simulink model "sm_DynamicCompressionOLD"  (R2019a)
settings: Solver=FixedStepDiscrete  StartTime=0.0  StopTime=stop_time  RelTol=1e-3
InitFcn:
  | sm_callback_init
StopFcn:
  | sm_callback_stop
values from neighbouring files (symbols this model uses):
  calib_bpfs = bpfs    [sm_compression_init.m]
  delayFix = maxDelay-delays    [Initialize_Delay_Values.m]
  F_bits = 28    [TestingLibraryScripts.m]    (also in sm_compression_init.m)
  M_bits = 1    [TestingLibraryScripts.m]    (also in sm_compression_init.m = 5)
  M_Bits = M_bits    (= 5)    [sm_compression_init.m]
  mp = sm_init_avalon_signals(mp)    [sm_callback_init.m]
  r_att = nthroot(0.1, s_att)    [sm_compression_init.m]
  r_rel = nthroot(0.1, s_rel)    [sm_compression_init.m]
  recombGain = ones(1,NChans)    [sm_compression_init.m]
  Ts = mp.Ts    [sm_compression_init.m]
  Ts_system = mp.Ts_system    [sm_compression_init.m]
  W_bits = 32    [TestingLibraryScripts.m]    (also in sm_compression_init.m)
  X_high = 1    [sm_compression_init.m]
undefined symbols (not defined in the file or in its folder): ig_eq, Table_Fill
libraries: simulink x355, hdlsllib x258, dsphdlfiltering x1
(part 1 of 7)
settings Model: Creator=Ross  LastModifiedBy=Bailey
settings DataIOCC: ReturnWorkspaceOutputs=off
settings OptimizationCC: BlockReduction=off  ConditionallyExecuteInputs=off  DefaultParameterBehavior=Inlined
settings DebuggingCC: ReadBeforeWriteMsg=DisableAll  WriteAfterWriteMsg=DisableAll  WriteAfterReadMsg=DisableAll  AlgebraicLoopMsg=error  MultiTaskDSMMsg=none  SingleTaskRateTransMsg=error  PregeneratedLibrarySubsystemCodeDiagnostic=none  ArithmeticOperatorsInVariantConditions=warning
settings HardwareCC: ProdBitPerPointer=32  ProdBitPerSizeT=32  ProdBitPerPtrDiffT=32  ProdLargestAtomicFloat=None  ProdIntDivRoundTo=Undefined  ProdEndianess=Unspecified  ProdWordSize=32  ProdHWDeviceType=ASIC/FPGA->ASIC/FPGA  TargetBitPerPointer=64  TargetBitPerSizeT=64  TargetBitPerPtrDiffT=64  TargetLongLongMode=on  TargetIntDivRoundTo=Zero  TargetEndianess=LittleEndian  TargetWordSize=64  TargetHWDeviceType=Custom Processor->MATLAB Host Computer  ProdEqTarget=off
settings ModelReferenceCC: UpdateModelReferenceTargets=IfOutOfDate
settings SFSimCC: SFSimEcho=off  SimUseLocalCustomCode=off
settings RTWCC: RTWUseLocalCustomCode=off

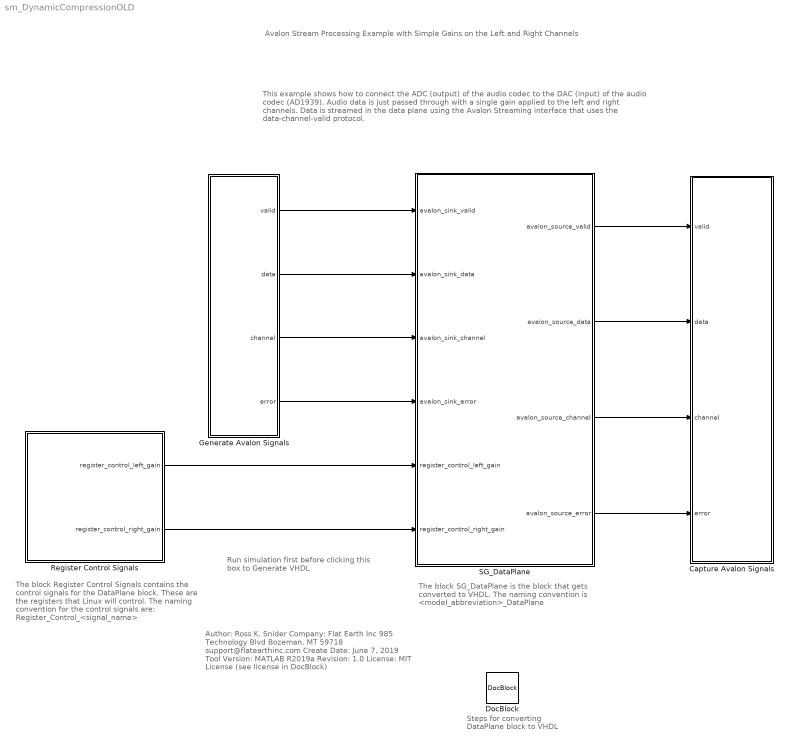
== system sm_DynamicCompressionOLD ==
  note: The block SG_DataPlane is the block that gets
      | converted to VHDL. The naming convention is
      | <model_abbreviation>_DataPlane
  note: Author:          Ross K. Snider
      | Company:     Flat Earth Inc
      |                       985 Technology Blvd
      |                       Bozeman, MT 59718
      |                       support@flatearthinc.com
      | Create Date:  June 7, 2019
      | Tool Version:  MATLAB R2019a
      | Revision:        1.0
      | License:          MIT License (see license in DocBlock)
  note: This example shows how to connect the ADC (output) of the audio codec to the DAC (input) of the audio codec (AD1939). Audio data is just passed through with a single gain applied to the left and right channels. Data is streamed in the data plane using the Avalon Streaming interface that uses the data-channel-valid protocol.
  note: Steps for converting
      | DataPlane block
      | to VHDL
  note: Avalon Stream Processing Example
      | with Simple Gains on the Left and Right Channels
  note: Run simulation first
      | before clicking this box to
      | Generate VHDL
  note: The block Register Control Signals contains
      | the control signals for the DataPlane block.
      | These are the registers that Linux will control.
      | The naming convention for the control
      | signals are:  Register_Control_<signal_name>
  Capture Avalon Signals : Subsystem
  DocBlock : simulink/Model-Wide Utilities/DocBlock  DocumentType=HTML
  Generate Avalon Signals : Subsystem
  Register Control Signals : Subsystem
  SG_DataPlane : Subsystem  TreatAsAtomicUnit=on
  wires:
  Generate Avalon Signals/2(data) -> SG_DataPlane/2(avalon_sink_data)
  Generate Avalon Signals/1(valid) -> SG_DataPlane/1(avalon_sink_valid)
  Generate Avalon Signals/3(channel) -> SG_DataPlane/3(avalon_sink_channel)
  Generate Avalon Signals/4(error) -> SG_DataPlane/4(avalon_sink_error)
  SG_DataPlane/2(avalon_source_data) -> Capture Avalon Signals/2(data)
  SG_DataPlane/1(avalon_source_valid) -> Capture Avalon Signals/1(valid)
  SG_DataPlane/3(avalon_source_channel) -> Capture Avalon Signals/3(channel)
  SG_DataPlane/4(avalon_source_error) -> Capture Avalon Signals/4(error)
  Register Control Signals/1(register_control_left_gain) -> SG_DataPlane/5(register_control_left_gain)
  Register Control Signals/2(register_control_right_gain) -> SG_DataPlane/6(register_control_right_gain)

== system sm_DynamicCompressionOLD/Capture Avalon Signals ==
  note: Note:  If these "To Workspace" variables show up under a variable called "out",
      | Open the Configure Logging... window (Simulation->Output->Configure Logging...)
      | and deselect the checkbox "Single simulation output:" found under the "Save to workspace or file" section.
  valid : Inport
  data : Inport  Port=2
  channel : Inport  Port=3
  error : Inport  Port=4
  To Workspace : ToWorkspace  VariableName=Avalon_Sink_Data  SaveFormat=Timeseries  SampleTime=-1
  To Workspace1 : ToWorkspace  VariableName=Avalon_Sink_Valid  SaveFormat=Timeseries  SampleTime=-1
  To Workspace2 : ToWorkspace  VariableName=Avalon_Sink_Channel  SaveFormat=Timeseries  SampleTime=-1
  To Workspace3 : ToWorkspace  VariableName=Avalon_Sink_Error  SaveFormat=Timeseries  SampleTime=-1
  wires:
  data/1 -> To Workspace/1
  valid/1 -> To Workspace1/1
  error/1 -> To Workspace3/1
  channel/1 -> To Workspace2/1

== system sm_DynamicCompressionOLD/Generate Avalon Signals ==
  note: Avalon Streaming Sink Signals
      | Note: We are assuming a specific system clock frequency that these signals are being clock in at.
      | The interface needs to be regenerated if this system clock frequency changes. Change system clock frequency in InitFcn callback in Model Explorer.
      |
      | -- Avalon streaming slave interface (sink)
      | AD1939_DAC_data : in std_logic_vector(31 downto 0); -- W=32; F=28; Signed 2's Complement
      | AD1939_DAC_channel : in std_logic_vector(1 downto 0); -- Left <-> channel 0; Right <-> channel 1 (other two channels are ignored)
      | AD1939_DAC_valid : in std_logic; -- asserted when data is valid
      | AD1939_DAC_error : in std_logic_vector(1 downto 0) -- error channel is ignored, assumed to be error free at this point
      |
      | For more information on the data-channel-valid protocol, s ee chapter 5 in Intel's Avalon Interfaced Specification (p. 40) at https://www.intel.com/content/dam/www/programmable/us/en/pdfs/literature/manual/mnl_avalon_spec.pdf
  Avalon Source Channel : FromWorkspace  VariableName=mp.Avalon_Source_Channel  OutDataTypeStr=double  SampleTime=mp.Ts_system
  "Avalon Source Data " : FromWorkspace  VariableName=mp.Avalon_Source_Data  OutDataTypeStr=double  SampleTime=mp.Ts_system
  Avalon Source Error : FromWorkspace  VariableName=mp.Avalon_Source_Error  OutDataTypeStr=double  SampleTime=mp.Ts_system
  Avalon Source Valid : FromWorkspace  VariableName=mp.Avalon_Source_Valid  OutDataTypeStr=double  SampleTime=mp.Ts_system
  Data Type Conversion : DataTypeConversion  OutDataTypeStr=fixdt(1,mp.W_bits,mp.F_bits)
  Data Type Conversion1 : DataTypeConversion  OutDataTypeStr=fixdt(0,2,0)
  Data Type Conversion2 : DataTypeConversion  OutDataTypeStr=boolean
  Data Type Conversion3 : DataTypeConversion  OutDataTypeStr=fixdt(0,2,0)
  valid : Outport
  data : Outport  Port=2
  channel : Outport  Port=3
  error : Outport  Port=4
  wires:
  Data Type Conversion1/1 -> channel/1
  Data Type Conversion2/1 -> valid/1
  Avalon Source Error/1 -> Data Type Conversion3/1
  Data Type Conversion/1 -> data/1
  Avalon Source Valid/1 -> Data Type Conversion2/1
  Data Type Conversion3/1 -> error/1
  Avalon Source Channel/1 -> Data Type Conversion1/1
  "Avalon Source Data "/1 -> Data Type Conversion/1

== system sm_DynamicCompressionOLD/Register Control Signals ==
  note: Control Signals that will be coming from Linux via
      | memory mapped registers need to have names
      | containing the prefix "register_control_"
      | (all lower case)
  Data Type Conversion1 : DataTypeConversion  OutDataTypeStr=fixdt(1,mp.W_bits,mp.F_bits)
  Data Type Conversion2 : DataTypeConversion  OutDataTypeStr=fixdt(1,mp.W_bits,mp.F_bits)
  Time Series Signal from Workspace 1 : FromWorkspace  VariableName=mp.register(1).timeseries  OutDataTypeStr=double  SampleTime=mp.Ts_system
  Time Series Signal from Workspace 2 : FromWorkspace  VariableName=mp.register(2).timeseries  OutDataTypeStr=double  SampleTime=mp.Ts_system
  register_control_left_gain : Outport
  register_control_right_gain : Outport  Port=2
  wires:
  Time Series Signal from Workspace 1/1 -> Data Type Conversion2/1
  Time Series Signal from Workspace 2/1 -> Data Type Conversion1/1
  Data Type Conversion2/1 -> register_control_left_gain/1
  Data Type Conversion1/1 -> register_control_right_gain/1

== system sm_DynamicCompressionOLD/SG_DataPlane ==
  note: Control Signals that will be coming from Linux via
      | memory mapped registers need to have names
      | containing the prefix "register_control_"
      | (all lower case)
  note: The Avalon Data Processing Block
      | performs DSP on the left and right channels.
  note: The Avalon Data Processing block
      | only executes when valid is asserted
  note: Ignore Errors.
      | Assuming no errors coming from the ADC and errors going to DAC will be ignored.
      | Any Error streaming needs to be done inside Avalon Data Processing block.
  note: Avalon streaming interface signals need to have the
      | names containing the prefix "avalon_"
      | (all lower case)
  avalon_sink_valid : Inport
  avalon_sink_data : Inport  Port=2
  avalon_sink_channel : Inport  Port=3
  avalon_sink_error : Inport  Port=4
  register_control_left_gain : Inport  Port=5
  register_control_right_gain : Inport  Port=6
  Avalon Data Processing : Subsystem  TreatAsAtomicUnit=on
  avalon_source_valid : Outport
  avalon_source_data : Outport  Port=2
  avalon_source_channel : Outport  Port=3
  avalon_source_error : Outport  Port=4
  wires:
  avalon_sink_channel/1 -> Avalon Data Processing/2(Sink_Channel)
  avalon_sink_error/1 -> avalon_source_error/1
  Avalon Data Processing/1(Source_Data) -> avalon_source_data/1
  avalon_sink_valid/1 -> avalon_source_valid/1, Avalon Data Processing/Enable
  avalon_sink_data/1 -> Avalon Data Processing/1(Sink_Data)
  Avalon Data Processing/2(Source_Channel) -> avalon_source_channel/1
  register_control_right_gain/1 -> Avalon Data Processing/4(Right_Gain)
  register_control_left_gain/1 -> Avalon Data Processing/3(Left_Gain)

== system sm_DynamicCompressionOLD/SG_DataPlane/Avalon Data Processing ==
  note: Select output data
      | based on channel number
  note: Check if Channel 0
      | (Left Channel)
  note: The Left Channel Processing block
      | only executes when channel 0
      | is detected
  note: The Right Channel Processing block
      | only executes when channel 1
      | is detected
  note: Check if Channel 1
      | (Right Channel)
  note: An enabled subsystem
      | This subsystem only runs when the data valid signal is enabled (asserted)
  Sink_Data : Inport
  Sink_Channel : Inport  Port=2
  Left_Gain : Inport  Port=3
  Right_Gain : Inport  Port=4
  Enable : EnablePort
  Compare To Constant1 : simulink/Logic and Bit Operations/Compare To Constant  relop===  const=1  OutDataTypeStr=boolean
  Compare To Constant2 : simulink/Logic and Bit Operations/Compare To Constant  relop===  const=0  OutDataTypeStr=boolean
  Left Channel Processing : Subsystem  TreatAsAtomicUnit=on
  Multiport Switch : MultiPortSwitch  DataPortOrder=Zero-based contiguous  zeroidx=on
  Right Channel Processing : Subsystem  TreatAsAtomicUnit=on
  Source_Data : Outport  InitialOutput=0
  Source_Channel : Outport  Port=2  InitialOutput=0
  wires:
  Sink_Channel/1 -> Source_Channel/1, Multiport Switch/1, Compare To Constant1/1, Compare To Constant2/1
  Compare To Constant2/1 -> Left Channel Processing/Enable
  Compare To Constant1/1 -> Right Channel Processing/Enable
  Sink_Data/1 -> Multiport Switch/4, Right Channel Processing/1(Right_Data_In), Left Channel Processing/1(Left_Data_In)
  Left Channel Processing/1("Left_Data_Out ") -> Multiport Switch/2
  Right Channel Processing/1("Right_Data_Out ") -> Multiport Switch/3
  Multiport Switch/1 -> Source_Data/1
  Left_Gain/1 -> Left Channel Processing/2(Left_Gain)
  Right_Gain/1 -> Right Channel Processing/2(Right_Gain)

== system sm_DynamicCompressionOLD/SG_DataPlane/Avalon Data Processing/Left Channel Processing ==
  note: An enabled subsystem
      | This subsystem only runs when the data valid signal is enabled (asserted)
  Left_Data_In : Inport
  Left_Gain : Inport  Port=2
  Enable : EnablePort
  Cast To Boolean : DataTypeConversion  OutDataTypeStr=boolean
  Cast To Boolean1 : DataTypeConversion  OutDataTypeStr=boolean
  Cast To fp(1,32,28) : DataTypeConversion  OutDataTypeStr=fixdt(1,32,28)  RndMeth=Round
  Cast To fp(1,32,28)1 : DataTypeConversion  OutDataTypeStr=fixdt(1,32,28)  RndMeth=Round
  From Workspace : FromWorkspace  VariableName=sig_in  SampleTime=Ts  OutputAfterFinalValue=Setting to zero
  From Workspace1 : FromWorkspace  VariableName=Table_Fill_t  SampleTime=Ts  Interpolate=off  OutputAfterFinalValue=Setting to zero
  From Workspace2 : FromWorkspace  VariableName=Fill_Valid_t  SampleTime=Ts  OutputAfterFinalValue=Setting to zero
  From Workspace4 : FromWorkspace  VariableName=Reset  SampleTime=Ts  Interpolate=off  OutputAfterFinalValue=Setting to zero
  Terminator : Terminator
  To Workspace : ToWorkspace  VariableName=proc_sig  SaveFormat=Timeseries  SampleTime=-1
  recalculate : Subsystem
  "Left_Data_Out " : Outport  InitialOutput=0
  wires:
  Cast To Boolean1/1 -> recalculate/4(Memory_Reset)
  Cast To Boolean/1 -> recalculate/2(Fill_Valid)
  Cast To fp(1,32,28)1/1 -> Terminator/1
  From Workspace1/1 -> Cast To fp(1,32,28)/1  "Table_Values"
  recalculate/1(proc_sig) -> To Workspace/1
  From Workspace2/1 -> Cast To Boolean/1
  From Workspace/1 -> Cast To fp(1,32,28)1/1
  From Workspace4/1 -> Cast To Boolean1/1
  Cast To fp(1,32,28)/1 -> recalculate/1(Table_Values)
  Left_Data_In/1 -> recalculate/3(sig)

== system sm_DynamicCompressionOLD/SG_DataPlane/Avalon Data Processing/Right Channel Processing ==
  note: Apply Right Gain
  note: An enabled subsystem
      | This subsystem only runs when the data valid signal is enabled (asserted)
  Right_Data_In : Inport
  Right_Gain : Inport  Port=2
  Enable : EnablePort
  Data Type Conversion : DataTypeConversion  OutDataTypeStr=fixdt(1,mp.W_bits,mp.F_bits)
  Product : Product
  "Right_Data_Out " : Outport  InitialOutput=0
  wires:
  Data Type Conversion/1 -> "Right_Data_Out "/1
  Product/1 -> Data Type Conversion/1
  Right_Data_In/1 -> Product/1
  Right_Gain/1 -> Product/2

== system sm_DynamicCompressionOLD/SG_DataPlane/Avalon Data Processing/Left Channel Processing/recalculate ==
  note: High Clipping
  note: Prescription Application
  note: Low Clipping
  Table_Values : Inport
  Fill_Valid : Inport  Port=2
  sig : Inport  Port=3
  Memory_Reset : Inport  Port=4
  Compare To Constant : simulink/Logic and Bit Operations/Compare To Constant  relop=>=  const=X_high  OutDataTypeStr=boolean
  Compare To Constant1 : simulink/Logic and Bit Operations/Compare To Constant  relop=<=  const=-X_high  OutDataTypeStr=boolean
  Constant : Constant  Value=X_high  OutDataTypeStr=fixdt(1,W_bits, F_bits)  SampleTime=-1
  Constant1 : Constant  Value=-X_high  OutDataTypeStr=fixdt(1,W_bits, F_bits)  SampleTime=-1
  Nchan_FbankAGC_AID : Subsystem
  Switch : Switch  Criteria=u2 ~= 0
  Switch1 : Switch  Criteria=u2 ~= 0
  ig65 fir : DiscreteFir  Coefficients=ig_eq  CoefDataTypeStr=fixdt(1, W_bits*2, W_bits)  ProductDataTypeStr=fixdt(1, W_bits*2, W_bits)  AccumDataTypeStr=fixdt(1, W_bits*2, W_bits)  OutDataTypeStr=fixdt(1, W_bits, F_bits)
  proc_sig : Outport
  wires:
  sig/1 -> Nchan_FbankAGC_AID/3(input_signal)
  Table_Values/1 -> Nchan_FbankAGC_AID/1(Table_Values)
  Fill_Valid/1 -> Nchan_FbankAGC_AID/2(Fill_Valid)
  Memory_Reset/1 -> Nchan_FbankAGC_AID/4(Reset)
  ig65 fir/1 -> Compare To Constant/1, Switch/3  "re_level.*eq_sig"
  Nchan_FbankAGC_AID/1(proc_sig) -> ig65 fir/1
  Compare To Constant/1 -> Switch/2
  Constant/1 -> Switch/1
  Switch/1 -> Switch1/3, Compare To Constant1/1
  Compare To Constant1/1 -> Switch1/2
  Constant1/1 -> Switch1/1
  Switch1/1 -> proc_sig/1

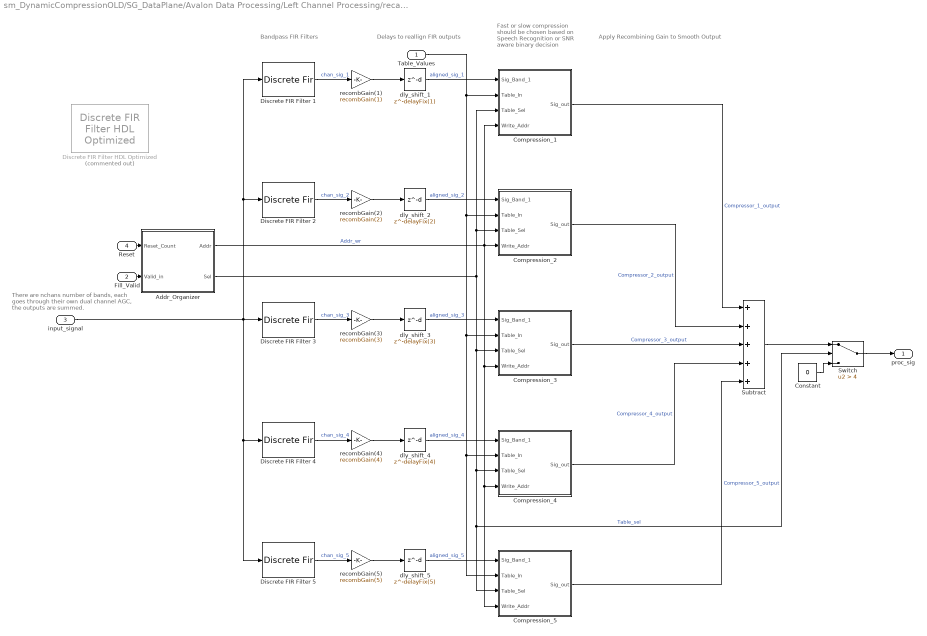
== system sm_DynamicCompressionOLD/SG_DataPlane/Avalon Data Processing/Left Channel Processing/recalculate/Nchan_FbankAGC_AID ==
  note: Apply Recombining Gain to Smooth Output
  note: Fast or slow compression
      | should be chosen based
      | on Speech Recognition or
      | SNR aware binary decision
  note: Delays to reallign FIR outputs
  note: Bandpass FIR Filters
  note: There are nchans number of bands,
      |  each goes through their own dual
      | channel AGC, the outputs are summed.
  Table_Values : Inport
  Fill_Valid : Inport  Port=2
  input_signal : Inport  Port=3
  Reset : Inport  Port=4
  Addr_Organizer : Subsystem
  Compression_1 : Subsystem
  Compression_2 : Subsystem
  Compression_3 : Subsystem
  Compression_4 : Subsystem
  Compression_5 : Subsystem
  Constant : Constant  Value=0  OutDataTypeStr=fixdt(1,W_bits, F_bits)  SampleTime=-1
  Discrete FIR Filter HDL Optimized : dsphdlfiltering/Discrete FIR Filter HDL Optimized  Commented=on  NumeratorSource=Property  Numerator=[ 0.5, 0.5 ]  NumeratorPrototype=[ 0.5, 0.5 ]  FilterStructure=Direct form systolic  SerializationOption=Minimum number of cycles between valid input samples  NumberOfCycles=2  NumberOfMultipliers=2  SimulateUsing=Code generation  roundingMode=Floor  overflowMode=off  CoefficientsDataTypeStr=Inherit: Same word length as input  CoefficientsMin=[]  CoefficientsMax=[]  OutputMin=[]  OutputMax=[]  ResetInputPort=off  HDLGlobalReset=off
      settings: SourceProductName=DSP System Toolbox  SourceProductBaseCode=DS
  Discrete FIR Filter 1 : DiscreteFir  Coefficients=calib_bpfs(2:calib_bpfs(1,1)+1 ,1)'  SampleTime=Ts  CoefDataTypeStr=fixdt(1, W_bits, F_bits)  ProductDataTypeStr=fixdt(1, W_bits, F_bits)  AccumDataTypeStr=fixdt(1, W_bits, F_bits)  OutDataTypeStr=fixdt(1, W_bits, F_bits)
  Discrete FIR Filter 2 : DiscreteFir  Coefficients=calib_bpfs(2:calib_bpfs(1,2)+1 ,2)'  CoefDataTypeStr=fixdt(1, W_bits, F_bits)  ProductDataTypeStr=fixdt(1, W_bits, F_bits)  AccumDataTypeStr=fixdt(1, W_bits, F_bits)  OutDataTypeStr=fixdt(1, W_bits, F_bits)
  Discrete FIR Filter 3 : DiscreteFir  Coefficients=calib_bpfs(2:calib_bpfs(1,3)+1 ,3)'  CoefDataTypeStr=fixdt(1, W_bits, F_bits)  ProductDataTypeStr=fixdt(1, W_bits, F_bits)  AccumDataTypeStr=fixdt(1, W_bits, F_bits)  OutDataTypeStr=fixdt(1, W_bits, F_bits)
  Discrete FIR Filter 4 : DiscreteFir  Coefficients=calib_bpfs(2:calib_bpfs(1,4)+1 ,4)'  CoefDataTypeStr=fixdt(1, W_bits, F_bits)  ProductDataTypeStr=fixdt(1, W_bits, F_bits)  AccumDataTypeStr=fixdt(1, W_bits, F_bits)  OutDataTypeStr=fixdt(1, W_bits, F_bits)
  Discrete FIR Filter 5 : DiscreteFir  Coefficients=calib_bpfs(2:calib_bpfs(1,5)+1 ,5)'  CoefDataTypeStr=fixdt(1, W_bits, F_bits)  ProductDataTypeStr=fixdt(1, W_bits, F_bits)  AccumDataTypeStr=fixdt(1, W_bits, F_bits)  OutDataTypeStr=fixdt(1, W_bits, F_bits)
  Subtract : Sum  Inputs=+++++
  Switch : Switch  Criteria=u2 > Threshold  Threshold=4
  dly_shift_1 : Delay  DelayLength=delayFix(1)  DelayLengthUpperLimit=500
  dly_shift_2 : Delay  DelayLength=delayFix(2)  DelayLengthUpperLimit=500
  dly_shift_3 : Delay  DelayLength=delayFix(3)  DelayLengthUpperLimit=500
  dly_shift_4 : Delay  DelayLength=delayFix(4)  DelayLengthUpperLimit=500
  dly_shift_5 : Delay  DelayLength=delayFix(5)  DelayLengthUpperLimit=500
  recombGain(1) : Gain  Gain=recombGain(1)  OutDataTypeStr=Inherit: Same as input
  recombGain(2) : Gain  Gain=recombGain(2)  OutDataTypeStr=Inherit: Same as input
  recombGain(3) : Gain  Gain=recombGain(3)  OutDataTypeStr=Inherit: Same as input
  recombGain(4) : Gain  Gain=recombGain(4)  OutDataTypeStr=Inherit: Same as input
  recombGain(5) : Gain  Gain=recombGain(5)  OutDataTypeStr=Inherit: Same as input
  proc_sig : Outport
  wires:
  Discrete FIR Filter 1/1 -> recombGain(1)/1  "chan_sig_1"
  dly_shift_1/1 -> Compression_1/1(Sig_Band_1)  "aligned_sig_1"
  Compression_1/1(Sig_out) -> Subtract/1  "Compressor_1_output"
  dly_shift_2/1 -> Compression_2/1(Sig_Band_1)  "aligned_sig_2"
  Discrete FIR Filter 2/1 -> recombGain(2)/1  "chan_sig_2"
  dly_shift_3/1 -> Compression_3/1(Sig_Band_1)  "aligned_sig_3"
  Discrete FIR Filter 3/1 -> recombGain(3)/1  "chan_sig_3"
  Discrete FIR Filter 5/1 -> recombGain(5)/1  "chan_sig_5"
  input_signal/1 -> Discrete FIR Filter 5/1, Discrete FIR Filter 4/1, Discrete FIR Filter 2/1, Discrete FIR Filter 1/1, Discrete FIR Filter 3/1
  dly_shift_5/1 -> Compression_5/1(Sig_Band_1)  "aligned_sig_5"
  dly_shift_4/1 -> Compression_4/1(Sig_Band_1)  "aligned_sig_4"
  Discrete FIR Filter 4/1 -> recombGain(4)/1  "chan_sig_4"
  Compression_3/1(Sig_out) -> Subtract/3  "Compressor_3_output"
  Compression_2/1(Sig_out) -> Subtract/2  "Compressor_2_output"
  Compression_4/1(Sig_out) -> Subtract/4  "Compressor_4_output"
  Compression_5/1(Sig_out) -> Subtract/5  "Compressor_5_output"
  Addr_Organizer/1(Addr) -> Compression_3/4(Write_Addr), Compression_5/4(Write_Addr), Compression_4/4(Write_Addr), Compression_2/4(Write_Addr), Compression_1/4(Write_Addr)  "Addr_wr"
  Reset/1 -> Addr_Organizer/1(Reset_Count)
  Fill_Valid/1 -> Addr_Organizer/2(Valid_in)
  Table_Values/1 -> Compression_5/2(Table_In), Compression_4/2(Table_In), Compression_3/2(Table_In), Compression_2/2(Table_In), Compression_1/2(Table_In)
  Addr_Organizer/2(Sel) -> Compression_3/3(Table_Sel), Compression_5/3(Table_Sel), Switch/2, Compression_4/3(Table_Sel), Compression_1/3(Table_Sel), Compression_2/3(Table_Sel)  "Table_sel"
  Subtract/1 -> Switch/1
  Constant/1 -> Switch/3
  Switch/1 -> proc_sig/1
  recombGain(1)/1 -> dly_shift_1/1
  recombGain(2)/1 -> dly_shift_2/1
  recombGain(3)/1 -> dly_shift_3/1
  recombGain(4)/1 -> dly_shift_4/1
  recombGain(5)/1 -> dly_shift_5/1

== system sm_DynamicCompressionOLD/SG_DataPlane/Avalon Data Processing/Left Channel Processing/recalculate/Nchan_FbankAGC_AID/Addr_Organizer ==
  note: Addr line contains the local address bits: 0-63
  note: Select Line is 000 to 101, if 110 writing is complete
  Reset_Count : Inport
  Valid_in : Inport  Port=2
  Bit Slice : hdlsllib/Logic and Bit Operations/Bit Slice  lidx=3+M_bits  ridx=0
      settings: SourceProductName=Simulink  SourceProductBaseCode=SL
  Bit Slice1 : hdlsllib/Logic and Bit Operations/Bit Slice  lidx=6+M_bits  ridx=4+M_bits
      settings: SourceProductName=Simulink  SourceProductBaseCode=SL
  Counter_up_to_320 : hdlsllib/Sources/HDL Counter  CountType=Count limited  CountInit=5*2^(4+M_Bits)  CountStep=1  CountMax=5*2^(4+M_Bits)+1  CountFromType=Initial value  CountFrom=5*2^(4+M_Bits)  CountResetPort=on  CountLoadPort=off  CountEnbPort=on  CountDirPort=off  CountDataType=Unsigned  CountWordLen=7+M_Bits  CountFracLen=0  CountSampTime=1
      settings: SourceProductName=Simulink
  Data Type Conversion : DataTypeConversion  OutDataTypeStr=fixdt(0,7+M_Bits,0)
  Data Type Conversion1 : DataTypeConversion  OutDataTypeStr=fixdt(0,4+M_bits,0)
  Data Type Conversion2 : DataTypeConversion  OutDataTypeStr=fixdt(0,3,0)
  Addr : Outport
  Sel : Outport  Port=2
  wires:
  Valid_in/1 -> Counter_up_to_320/2
  Reset_Count/1 -> Counter_up_to_320/1
  Counter_up_to_320/1 -> Data Type Conversion/1
  Data Type Conversion/1 -> Bit Slice1/1, Bit Slice/1
  Bit Slice1/1 -> Data Type Conversion2/1  "top3Bits"
  Bit Slice/1 -> Data Type Conversion1/1
  Data Type Conversion1/1 -> Addr/1
  Data Type Conversion2/1 -> Sel/1

== system sm_DynamicCompressionOLD/SG_DataPlane/Avalon Data Processing/Left Channel Processing/recalculate/Nchan_FbankAGC_AID/Compression_1 ==
  note: Calculate Compression Gain Needed
  note: Apply to the Envelope
  Sig_Band_1 : Inport
  Table_In : Inport  Port=2
  Table_Sel : Inport  Port=3
  Write_Addr : Inport  Port=4
  Compare To Constant : simulink/Logic and Bit Operations/Compare To Constant  relop===  const=0  OutDataTypeStr=boolean
  Compression_Envelope : Subsystem
  Compression_Gain_Calc : Subsystem
  Constant : Constant  Value=0  OutDataTypeStr=fixdt(1,W_bits,F_bits)  SampleTime=-1
  Data Type Conversion1 : DataTypeConversion  OutDataTypeStr=fixdt(1,W_bits,F_bits)
  Delay : Delay  DelayLength=3
  Product : Product
  Switch : Switch  Criteria=u2 > Threshold  Threshold=4  ZeroCross=off
  Unit Delay : UnitDelay  InitialCondition=1  SampleTime=-1  HasFrameUpgradeWarning=on
  Sig_out : Outport
  wires:
  Compression_Envelope/1(Gain_Out) -> Product/1, Unit Delay/1
  Unit Delay/1 -> Compression_Envelope/2(Curr_Gain)
  Product/1 -> Data Type Conversion1/1
  Compare To Constant/1 -> Compression_Gain_Calc/3(Table_Fill_Valid)
  Write_Addr/1 -> Compression_Gain_Calc/2(Write_Addr)
  Table_In/1 -> Compression_Gain_Calc/1(Table_Fill)  "Table_Values"
  Switch/1 -> Delay/1
  Table_Sel/1 -> Compare To Constant/1, Switch/2
  Constant/1 -> Switch/3
  Sig_Band_1/1 -> Compression_Gain_Calc/4(Data_In), Switch/1
  Data Type Conversion1/1 -> Sig_out/1
  Delay/1 -> Product/2
  Compression_Gain_Calc/1(Gain_C_out) -> Compression_Envelope/1(Desired_Gain)

== system sm_DynamicCompressionOLD/SG_DataPlane/Avalon Data Processing/Left Channel Processing/recalculate/Nchan_FbankAGC_AID/Compression_2 ==
  note: Calculate Compression Gain Needed
  note: Apply to the Envelope
  Sig_Band_1 : Inport
  Table_In : Inport  Port=2
  Table_Sel : Inport  Port=3
  Write_Addr : Inport  Port=4
  Compare To Constant : simulink/Logic and Bit Operations/Compare To Constant  relop===  const=1  OutDataTypeStr=boolean
  Compression_Envelope : Subsystem
  Compression_Gain_Calc : Subsystem
  Constant : Constant  Value=0  OutDataTypeStr=fixdt(1,W_bits,F_bits)  SampleTime=-1
  Data Type Conversion1 : DataTypeConversion  OutDataTypeStr=fixdt(1,W_bits,F_bits)
  Delay : Delay  DelayLength=3
  Product : Product
  Switch : Switch  Criteria=u2 > Threshold  Threshold=4  ZeroCross=off
  Unit Delay : UnitDelay  InitialCondition=1  SampleTime=-1  HasFrameUpgradeWarning=on
  Sig_out : Outport
  wires:
  Compression_Envelope/1(Gain_Out) -> Product/1, Unit Delay/1
  Unit Delay/1 -> Compression_Envelope/2(Curr_Gain)
  Compare To Constant/1 -> Compression_Gain_Calc/3(Table_Fill_Valid)
  Write_Addr/1 -> Compression_Gain_Calc/2(Write_Addr)
  Table_In/1 -> Compression_Gain_Calc/1(Table_Fill)  "Table_Values"
  Table_Sel/1 -> Compare To Constant/1, Switch/2
  Constant/1 -> Switch/3
  Switch/1 -> Delay/1
  Sig_Band_1/1 -> Compression_Gain_Calc/4(Data_In), Switch/1
  Product/1 -> Data Type Conversion1/1
  Data Type Conversion1/1 -> Sig_out/1
  Delay/1 -> Product/2
  Compression_Gain_Calc/1(Gain_C_out) -> Compression_Envelope/1(Desired_Gain)

== system sm_DynamicCompressionOLD/SG_DataPlane/Avalon Data Processing/Left Channel Processing/recalculate/Nchan_FbankAGC_AID/Compression_3 ==
  note: Calculate Compression Gain Needed
  note: Apply to the Envelope
  Sig_Band_1 : Inport
  Table_In : Inport  Port=2
  Table_Sel : Inport  Port=3
  Write_Addr : Inport  Port=4
  Compare To Constant : simulink/Logic and Bit Operations/Compare To Constant  relop===  const=2  OutDataTypeStr=boolean
  Compression_Envelope : Subsystem
  Compression_Gain_Calc : Subsystem
  Constant : Constant  Value=0  OutDataTypeStr=fixdt(1,W_bits,F_bits)  SampleTime=-1
  Data Type Conversion1 : DataTypeConversion  OutDataTypeStr=fixdt(1,W_bits,F_bits)
  Delay : Delay  DelayLength=3
  Product : Product
  Switch : Switch  Criteria=u2 > Threshold  Threshold=4  ZeroCross=off
  Unit Delay : UnitDelay  InitialCondition=1  SampleTime=-1  HasFrameUpgradeWarning=on
  Sig_out : Outport
  wires:
  Compression_Envelope/1(Gain_Out) -> Product/1, Unit Delay/1
  Unit Delay/1 -> Compression_Envelope/2(Curr_Gain)
  Compare To Constant/1 -> Compression_Gain_Calc/3(Table_Fill_Valid)
  Write_Addr/1 -> Compression_Gain_Calc/2(Write_Addr)
  Table_In/1 -> Compression_Gain_Calc/1(Table_Fill)  "Table_Values"
  Switch/1 -> Delay/1
  Table_Sel/1 -> Compare To Constant/1, Switch/2
  Constant/1 -> Switch/3
  Sig_Band_1/1 -> Compression_Gain_Calc/4(Data_In), Switch/1
  Product/1 -> Data Type Conversion1/1
  Data Type Conversion1/1 -> Sig_out/1
  Delay/1 -> Product/2
  Compression_Gain_Calc/1(Gain_C_out) -> Compression_Envelope/1(Desired_Gain)

== system sm_DynamicCompressionOLD/SG_DataPlane/Avalon Data Processing/Left Channel Processing/recalculate/Nchan_FbankAGC_AID/Compression_4 ==
  note: Calculate Compression Gain Needed
  note: Apply to the Envelope
  Sig_Band_1 : Inport
  Table_In : Inport  Port=2
  Table_Sel : Inport  Port=3
  Write_Addr : Inport  Port=4
  Compare To Constant : simulink/Logic and Bit Operations/Compare To Constant  relop===  const=3  OutDataTypeStr=boolean
  Compression_Envelope : Subsystem
  Compression_Gain_Calc : Subsystem
  Constant : Constant  Value=0  OutDataTypeStr=fixdt(1,W_bits,F_bits)  SampleTime=-1
  Data Type Conversion1 : DataTypeConversion  OutDataTypeStr=fixdt(1,W_bits,F_bits)
  Delay : Delay  DelayLength=3
  Product : Product
  Switch : Switch  Criteria=u2 > Threshold  Threshold=4  ZeroCross=off
  Unit Delay : UnitDelay  InitialCondition=1  SampleTime=-1  HasFrameUpgradeWarning=on
  Sig_out : Outport
  wires:
  Compression_Envelope/1(Gain_Out) -> Product/1, Unit Delay/1
  Unit Delay/1 -> Compression_Envelope/2(Curr_Gain)
  Compare To Constant/1 -> Compression_Gain_Calc/3(Table_Fill_Valid)
  Compression_Gain_Calc/1(Gain_C_out) -> Compression_Envelope/1(Desired_Gain)
  Write_Addr/1 -> Compression_Gain_Calc/2(Write_Addr)
  Table_In/1 -> Compression_Gain_Calc/1(Table_Fill)  "Table_Values"
  Switch/1 -> Delay/1
  Table_Sel/1 -> Compare To Constant/1, Switch/2
  Constant/1 -> Switch/3
  Sig_Band_1/1 -> Compression_Gain_Calc/4(Data_In), Switch/1
  Product/1 -> Data Type Conversion1/1
  Data Type Conversion1/1 -> Sig_out/1
  Delay/1 -> Product/2

== system sm_DynamicCompressionOLD/SG_DataPlane/Avalon Data Processing/Left Channel Processing/recalculate/Nchan_FbankAGC_AID/Compression_5 ==
  note: Calculate Compression Gain Needed
  note: Apply to the Envelope
  Sig_Band_1 : Inport
  Table_In : Inport  Port=2
  Table_Sel : Inport  Port=3
  Write_Addr : Inport  Port=4
  Compare To Constant : simulink/Logic and Bit Operations/Compare To Constant  relop===  const=4  OutDataTypeStr=boolean
  Compression_Envelope : Subsystem
  Compression_Gain_Calc : Subsystem
  Constant : Constant  Value=0  OutDataTypeStr=fixdt(1,W_bits,F_bits)  SampleTime=-1
  Data Type Conversion1 : DataTypeConversion  OutDataTypeStr=fixdt(1,W_bits,F_bits)
  Delay : Delay  DelayLength=3
  Product : Product
  Switch : Switch  Criteria=u2 > Threshold  Threshold=4  ZeroCross=off
  Unit Delay : UnitDelay  InitialCondition=1  SampleTime=-1  HasFrameUpgradeWarning=on
  Sig_out : Outport
  wires:
  Compression_Envelope/1(Gain_Out) -> Product/1, Unit Delay/1
  Unit Delay/1 -> Compression_Envelope/2(Curr_Gain)
  Compare To Constant/1 -> Compression_Gain_Calc/3(Table_Fill_Valid)
  Compression_Gain_Calc/1(Gain_C_out) -> Compression_Envelope/1(Desired_Gain)
  Write_Addr/1 -> Compression_Gain_Calc/2(Write_Addr)
  Table_In/1 -> Compression_Gain_Calc/1(Table_Fill)  "Table_Values"
  Switch/1 -> Delay/1
  Table_Sel/1 -> Compare To Constant/1, Switch/2
  Constant/1 -> Switch/3
  Sig_Band_1/1 -> Compression_Gain_Calc/4(Data_In), Switch/1
  Product/1 -> Data Type Conversion1/1
  Data Type Conversion1/1 -> Sig_out/1
  Delay/1 -> Product/2

== system sm_DynamicCompressionOLD/SG_DataPlane/Avalon Data Processing/Left Channel Processing/recalculate/Nchan_FbankAGC_AID/Compression_1/Compression_Envelope ==
  note: Curr > Desired:
      | Attack
  note: Curr < Desired:
      | Release
  Desired_Gain : Inport
  Curr_Gain : Inport  Port=2
  Attack_Envelope : Subsystem  TreatAsAtomicUnit=on
  Compare To Zero : simulink/Logic and Bit Operations/Compare To Zero  relop=>=  OutDataTypeStr=boolean
  Logical Operator : Logic  Operator=NOT  AllPortsSameDT=off  OutDataTypeStr=boolean
  Release_Envelope : Subsystem  TreatAsAtomicUnit=on
  Subtract : Sum  Inputs=-+  AccumDataTypeStr=fixdt(1,W_bits,F_bits)  OutDataTypeStr=Inherit: Same as accumulator
  Switch : Switch
  Gain_Out : Outport
  wires:
  Desired_Gain/1 -> Attack_Envelope/2(Desired), Release_Envelope/2(Desired), Subtract/1
  Curr_Gain/1 -> Attack_Envelope/1(Curr), Subtract/2, Release_Envelope/1(Curr)
  Subtract/1 -> Switch/2, Compare To Zero/1
  Compare To Zero/1 -> Attack_Envelope/Enable, Logical Operator/1
  Logical Operator/1 -> Release_Envelope/Enable
  Switch/1 -> Gain_Out/1
  Attack_Envelope/1(Gain_out) -> Switch/1
  Release_Envelope/1(Gain_out) -> Switch/3

== system sm_DynamicCompressionOLD/SG_DataPlane/Avalon Data Processing/Left Channel Processing/recalculate/Nchan_FbankAGC_AID/Compression_1/Compression_Gain_Calc ==
  note: Data_In assumed before applied prescription FIR
  note: Compression: Assume the input is a single band coming from the system.
      |
      | Goals:
      | 	- Take in a single point
      | 	- compare the volume to a known hard cap for the data
      | 	- attenuate the signal if it's above a certain threshold
      | 		- the distance above the threshold should be cut in dB by a ratio R
      | 	- return the output point at the same sample rate received
  Table_Fill : Inport
  Write_Addr : Inport  Port=2
  Table_Fill_Valid : Inport  Port=3
  Data_In : Inport  Port=4
  Abs : Abs
  Constant : Constant  OutDataTypeStr=fixdt(0,9,0)  SampleTime=-1
  High_Gain_Table : Subsystem  AncestorBlock=hdlsllibUNLOCKED/HDL RAMs/Dual Port RAM  mask(Dual-port RAM){ram_size=4+M_Bits}
      mask prompts: ram_size "Address port width (2 to 29 bits)"
      mask help: This block simulates a dual-port RAM with two data output ports.
      mask init:
      | hdlblkmask_dpram;
      mask Help: helpview([docroot '/simulink/helptargets.map'],'HDL_dual_port_RAM');
  Linear_Approximation : Subsystem
  LogAddressing : Subsystem
  Low_Gain_Table : Subsystem  mask(Dual-port RAM){ram_size=4+M_Bits}
      mask prompts: ram_size "Address port width (2 to 29 bits)"
      mask help: This block simulates a dual-port RAM with two data output ports.
      mask init:
      | hdlblkmask_dpram;
      mask Help: helpview([docroot '/simulink/helptargets.map'],'HDL_dual_port_RAM');
  Subtract : Sum  OutDataTypeStr=Inherit: Same as first input
  Terminator : Terminator
  Terminator1 : Terminator
  Unit Delay1 : UnitDelay  InitialCondition=1  SampleTime=-1  HasFrameUpgradeWarning=on
  Unit Delay2 : UnitDelay  InitialCondition=1  SampleTime=-1  HasFrameUpgradeWarning=on
  Unit Delay3 : UnitDelay  InitialCondition=1  SampleTime=-1  HasFrameUpgradeWarning=on
  Gain_C_out : Outport
  wires:
  Table_Fill/1 -> High_Gain_Table/1(wr_din), Low_Gain_Table/1(wr_din)
  Table_Fill_Valid/1 -> High_Gain_Table/3(wr_en), Low_Gain_Table/3(wr_en)
  Write_Addr/1 -> High_Gain_Table/2(wr_addr), Low_Gain_Table/2(wr_addr)
  LogAddressing/1(addr_r) -> Low_Gain_Table/4(rd_addr), Unit Delay3/1, Subtract/1  "addr_low"
  Abs/1 -> Unit Delay2/1, LogAddressing/1(x_in)  "|X_in|"
  Data_In/1 -> Abs/1
  Constant/1 -> Subtract/2
  Subtract/1 -> High_Gain_Table/4(rd_addr)  "addr_high"
  Low_Gain_Table/1(wr_dout) -> Terminator/1
  High_Gain_Table/1(wr_dout) -> Terminator1/1
  High_Gain_Table/2(rd_dout) -> Linear_Approximation/1(G_high)  "G_high"
  Low_Gain_Table/2(rd_dout) -> Linear_Approximation/2(G_low)  "G_low"
  Linear_Approximation/1(G_Desired) -> Gain_C_out/1
  Unit Delay2/1 -> Unit Delay1/1
  Unit Delay1/1 -> Linear_Approximation/4(|X_in|)
  Unit Delay3/1 -> Linear_Approximation/3(addr_low)

== system sm_DynamicCompressionOLD/SG_DataPlane/Avalon Data Processing/Left Channel Processing/recalculate/Nchan_FbankAGC_AID/Compression_2/Compression_Envelope ==
  note: Curr > Desired:
      | Attack
  note: Curr < Desired:
      | Release
  Desired_Gain : Inport
  Curr_Gain : Inport  Port=2
  Attack_Envelope : Subsystem  TreatAsAtomicUnit=on
  Compare To Zero : simulink/Logic and Bit Operations/Compare To Zero  relop=>=  OutDataTypeStr=boolean
  Logical Operator : Logic  Operator=NOT  AllPortsSameDT=off  OutDataTypeStr=boolean
  Release_Envelope : Subsystem  TreatAsAtomicUnit=on
  Subtract : Sum  Inputs=-+  AccumDataTypeStr=fixdt(1,W_bits,F_bits)  OutDataTypeStr=Inherit: Same as accumulator
  Switch : Switch
  Gain_Out : Outport
  wires:
  Desired_Gain/1 -> Attack_Envelope/2(Desired), Release_Envelope/2(Desired), Subtract/1
  Curr_Gain/1 -> Attack_Envelope/1(Curr), Subtract/2, Release_Envelope/1(Curr)
  Subtract/1 -> Switch/2, Compare To Zero/1
  Compare To Zero/1 -> Attack_Envelope/Enable, Logical Operator/1
  Logical Operator/1 -> Release_Envelope/Enable
  Switch/1 -> Gain_Out/1
  Attack_Envelope/1(Gain_out) -> Switch/1
  Release_Envelope/1(Gain_out) -> Switch/3

== system sm_DynamicCompressionOLD/SG_DataPlane/Avalon Data Processing/Left Channel Processing/recalculate/Nchan_FbankAGC_AID/Compression_2/Compression_Gain_Calc ==
  note: Data_In assumed before applied prescription FIR
  note: Compression: Assume the input is a single band coming from the system.
      |
      | Goals:
      | 	- Take in a single point
      | 	- compare the volume to a known hard cap for the data
      | 	- attenuate the signal if it's above a certain threshold
      | 		- the distance above the threshold should be cut in dB by a ratio R
      | 	- return the output point at the same sample rate received
  Table_Fill : Inport
  Write_Addr : Inport  Port=2
  Table_Fill_Valid : Inport  Port=3
  Data_In : Inport  Port=4
  Abs : Abs
  Constant : Constant  OutDataTypeStr=fixdt(0,9,0)  SampleTime=-1
  High_Gain_Table : Subsystem  AncestorBlock=hdlsllibUNLOCKED/HDL RAMs/Dual Port RAM  mask(Dual-port RAM){ram_size=4+M_Bits}
      mask prompts: ram_size "Address port width (2 to 29 bits)"
      mask help: This block simulates a dual-port RAM with two data output ports.
      mask init:
      | hdlblkmask_dpram;
      mask Help: helpview([docroot '/simulink/helptargets.map'],'HDL_dual_port_RAM');
  Linear_Approximation : Subsystem
  LogAddressing : Subsystem
  Low_Gain_Table : Subsystem  AncestorBlock=hdlsllibUNLOCKED/HDL RAMs/Dual Port RAM  mask(Dual-port RAM){ram_size=4+M_Bits}
      mask prompts: ram_size "Address port width (2 to 29 bits)"
      mask help: This block simulates a dual-port RAM with two data output ports.
      mask init:
      | hdlblkmask_dpram;
      mask Help: helpview([docroot '/simulink/helptargets.map'],'HDL_dual_port_RAM');
  Subtract : Sum  OutDataTypeStr=Inherit: Same as first input
  Terminator : Terminator
  Terminator1 : Terminator
  Unit Delay1 : UnitDelay  InitialCondition=1  SampleTime=-1  HasFrameUpgradeWarning=on
  Unit Delay2 : UnitDelay  InitialCondition=1  SampleTime=-1  HasFrameUpgradeWarning=on
  Unit Delay3 : UnitDelay  InitialCondition=1  SampleTime=-1  HasFrameUpgradeWarning=on
  Gain_C_out : Outport
  wires:
  Table_Fill/1 -> High_Gain_Table/1(wr_din), Low_Gain_Table/1(wr_din)
  Table_Fill_Valid/1 -> High_Gain_Table/3(wr_en), Low_Gain_Table/3(wr_en)
  Write_Addr/1 -> High_Gain_Table/2(wr_addr), Low_Gain_Table/2(wr_addr)
  LogAddressing/1(addr_r) -> Low_Gain_Table/4(rd_addr), Unit Delay3/1, Subtract/1  "addr_low"
  Abs/1 -> Unit Delay2/1, LogAddressing/1(x_in)  "|X_in|"
  Data_In/1 -> Abs/1
  Constant/1 -> Subtract/2
  Subtract/1 -> High_Gain_Table/4(rd_addr)  "addr_high"
  Low_Gain_Table/1(wr_dout) -> Terminator/1
  High_Gain_Table/1(wr_dout) -> Terminator1/1
  High_Gain_Table/2(rd_dout) -> Linear_Approximation/1(G_high)  "G_high"
  Low_Gain_Table/2(rd_dout) -> Linear_Approximation/2(G_low)  "G_low"
  Linear_Approximation/1(G_Desired) -> Gain_C_out/1
  Unit Delay2/1 -> Unit Delay1/1
  Unit Delay1/1 -> Linear_Approximation/4(|X_in|)
  Unit Delay3/1 -> Linear_Approximation/3(addr_low)

== system sm_DynamicCompressionOLD/SG_DataPlane/Avalon Data Processing/Left Channel Processing/recalculate/Nchan_FbankAGC_AID/Compression_3/Compression_Envelope ==
  note: Curr > Desired:
      | Attack
  note: Curr < Desired:
      | Release
  Desired_Gain : Inport
  Curr_Gain : Inport  Port=2
  Attack_Envelope : Subsystem  TreatAsAtomicUnit=on
  Compare To Zero : simulink/Logic and Bit Operations/Compare To Zero  relop=>=  OutDataTypeStr=boolean
  Logical Operator : Logic  Operator=NOT  AllPortsSameDT=off  OutDataTypeStr=boolean
  Release_Envelope : Subsystem  TreatAsAtomicUnit=on
  Subtract : Sum  Inputs=-+  AccumDataTypeStr=fixdt(1,W_bits,F_bits)  OutDataTypeStr=Inherit: Same as accumulator
  Switch : Switch
  Gain_Out : Outport
  wires:
  Desired_Gain/1 -> Attack_Envelope/2(Desired), Release_Envelope/2(Desired), Subtract/1
  Curr_Gain/1 -> Attack_Envelope/1(Curr), Subtract/2, Release_Envelope/1(Curr)
  Subtract/1 -> Switch/2, Compare To Zero/1
  Compare To Zero/1 -> Attack_Envelope/Enable, Logical Operator/1
  Logical Operator/1 -> Release_Envelope/Enable
  Switch/1 -> Gain_Out/1
  Attack_Envelope/1(Gain_out) -> Switch/1
  Release_Envelope/1(Gain_out) -> Switch/3

== system sm_DynamicCompressionOLD/SG_DataPlane/Avalon Data Processing/Left Channel Processing/recalculate/Nchan_FbankAGC_AID/Compression_3/Compression_Gain_Calc ==
  note: Data_In assumed before applied prescription FIR
  note: Compression: Assume the input is a single band coming from the system.
      |
      | Goals:
      | 	- Take in a single point
      | 	- compare the volume to a known hard cap for the data
      | 	- attenuate the signal if it's above a certain threshold
      | 		- the distance above the threshold should be cut in dB by a ratio R
      | 	- return the output point at the same sample rate received
  Table_Fill : Inport
  Write_Addr : Inport  Port=2
  Table_Fill_Valid : Inport  Port=3
  Data_In : Inport  Port=4
  Abs : Abs
  Constant : Constant  OutDataTypeStr=fixdt(0,9,0)  SampleTime=-1
  High_Gain_Table : Subsystem  AncestorBlock=hdlsllibUNLOCKED/HDL RAMs/Dual Port RAM  mask(Dual-port RAM){ram_size=4+M_Bits}
      mask prompts: ram_size "Address port width (2 to 29 bits)"
      mask help: This block simulates a dual-port RAM with two data output ports.
      mask init:
      | hdlblkmask_dpram;
      mask Help: helpview([docroot '/simulink/helptargets.map'],'HDL_dual_port_RAM');
  Linear_Approximation : Subsystem
  LogAddressing : Subsystem
  Low_Gain_Table : Subsystem  AncestorBlock=hdlsllibUNLOCKED/HDL RAMs/Dual Port RAM  mask(Dual-port RAM){ram_size=4+M_Bits}
      mask prompts: ram_size "Address port width (2 to 29 bits)"
      mask help: This block simulates a dual-port RAM with two data output ports.
      mask init:
      | hdlblkmask_dpram;
      mask Help: helpview([docroot '/simulink/helptargets.map'],'HDL_dual_port_RAM');
  Subtract : Sum  OutDataTypeStr=Inherit: Same as first input
  Terminator : Terminator
  Terminator1 : Terminator
  Unit Delay1 : UnitDelay  InitialCondition=1  SampleTime=-1  HasFrameUpgradeWarning=on
  Unit Delay2 : UnitDelay  InitialCondition=1  SampleTime=-1  HasFrameUpgradeWarning=on
  Unit Delay3 : UnitDelay  InitialCondition=1  SampleTime=-1  HasFrameUpgradeWarning=on
  Gain_C_out : Outport
  wires:
  Table_Fill/1 -> High_Gain_Table/1(wr_din), Low_Gain_Table/1(wr_din)
  Table_Fill_Valid/1 -> High_Gain_Table/3(wr_en), Low_Gain_Table/3(wr_en)
  Write_Addr/1 -> High_Gain_Table/2(wr_addr), Low_Gain_Table/2(wr_addr)
  LogAddressing/1(addr_r) -> Low_Gain_Table/4(rd_addr), Unit Delay3/1, Subtract/1  "addr_low"
  Abs/1 -> Unit Delay2/1, LogAddressing/1(x_in)  "|X_in|"
  Data_In/1 -> Abs/1
  Constant/1 -> Subtract/2
  Subtract/1 -> High_Gain_Table/4(rd_addr)  "addr_high"
  Low_Gain_Table/1(wr_dout) -> Terminator/1
  High_Gain_Table/1(wr_dout) -> Terminator1/1
  High_Gain_Table/2(rd_dout) -> Linear_Approximation/1(G_high)  "G_high"
  Low_Gain_Table/2(rd_dout) -> Linear_Approximation/2(G_low)  "G_low"
  Linear_Approximation/1(G_Desired) -> Gain_C_out/1
  Unit Delay2/1 -> Unit Delay1/1
  Unit Delay1/1 -> Linear_Approximation/4(|X_in|)
  Unit Delay3/1 -> Linear_Approximation/3(addr_low)

== system sm_DynamicCompressionOLD/SG_DataPlane/Avalon Data Processing/Left Channel Processing/recalculate/Nchan_FbankAGC_AID/Compression_4/Compression_Envelope ==
  note: Curr > Desired:
      | Attack
  note: Curr < Desired:
      | Release
  Desired_Gain : Inport
  Curr_Gain : Inport  Port=2
  Attack_Envelope : Subsystem  TreatAsAtomicUnit=on
  Compare To Zero : simulink/Logic and Bit Operations/Compare To Zero  relop=>=  OutDataTypeStr=boolean
  Logical Operator : Logic  Operator=NOT  AllPortsSameDT=off  OutDataTypeStr=boolean
  Release_Envelope : Subsystem  TreatAsAtomicUnit=on
  Subtract : Sum  Inputs=-+  AccumDataTypeStr=fixdt(1,W_bits,F_bits)  OutDataTypeStr=Inherit: Same as accumulator
  Switch : Switch
  Gain_Out : Outport
  wires:
  Desired_Gain/1 -> Attack_Envelope/2(Desired), Release_Envelope/2(Desired), Subtract/1
  Curr_Gain/1 -> Attack_Envelope/1(Curr), Subtract/2, Release_Envelope/1(Curr)
  Subtract/1 -> Switch/2, Compare To Zero/1
  Compare To Zero/1 -> Attack_Envelope/Enable, Logical Operator/1
  Logical Operator/1 -> Release_Envelope/Enable
  Switch/1 -> Gain_Out/1
  Attack_Envelope/1(Gain_out) -> Switch/1
  Release_Envelope/1(Gain_out) -> Switch/3

== system sm_DynamicCompressionOLD/SG_DataPlane/Avalon Data Processing/Left Channel Processing/recalculate/Nchan_FbankAGC_AID/Compression_4/Compression_Gain_Calc ==
  note: Data_In assumed before applied prescription FIR
  note: Compression: Assume the input is a single band coming from the system.
      |
      | Goals:
      | 	- Take in a single point
      | 	- compare the volume to a known hard cap for the data
      | 	- attenuate the signal if it's above a certain threshold
      | 		- the distance above the threshold should be cut in dB by a ratio R
      | 	- return the output point at the same sample rate received
  Table_Fill : Inport
  Write_Addr : Inport  Port=2
  Table_Fill_Valid : Inport  Port=3
  Data_In : Inport  Port=4
  Abs : Abs
  Constant : Constant  OutDataTypeStr=fixdt(0,9,0)  SampleTime=-1
  High_Gain_Table : Subsystem  AncestorBlock=hdlsllibUNLOCKED/HDL RAMs/Dual Port RAM  mask(Dual-port RAM){ram_size=4+M_Bits}
      mask prompts: ram_size "Address port width (2 to 29 bits)"
      mask help: This block simulates a dual-port RAM with two data output ports.
      mask init:
      | hdlblkmask_dpram;
      mask Help: helpview([docroot '/simulink/helptargets.map'],'HDL_dual_port_RAM');
  Linear_Approximation : Subsystem
  LogAddressing : Subsystem
  Low_Gain_Table : Subsystem  AncestorBlock=hdlsllibUNLOCKED/HDL RAMs/Dual Port RAM  mask(Dual-port RAM){ram_size=4+M_Bits}
      mask prompts: ram_size "Address port width (2 to 29 bits)"
      mask help: This block simulates a dual-port RAM with two data output ports.
      mask init:
      | hdlblkmask_dpram;
      mask Help: helpview([docroot '/simulink/helptargets.map'],'HDL_dual_port_RAM');
  Subtract : Sum  OutDataTypeStr=Inherit: Same as first input
  Terminator : Terminator
  Terminator1 : Terminator
  Unit Delay1 : UnitDelay  InitialCondition=1  SampleTime=-1  HasFrameUpgradeWarning=on
  Unit Delay2 : UnitDelay  InitialCondition=1  SampleTime=-1  HasFrameUpgradeWarning=on
  Unit Delay3 : UnitDelay  InitialCondition=1  SampleTime=-1  HasFrameUpgradeWarning=on
  Gain_C_out : Outport
  wires:
  Table_Fill/1 -> High_Gain_Table/1(wr_din), Low_Gain_Table/1(wr_din)
  Table_Fill_Valid/1 -> High_Gain_Table/3(wr_en), Low_Gain_Table/3(wr_en)
  Write_Addr/1 -> High_Gain_Table/2(wr_addr), Low_Gain_Table/2(wr_addr)
  LogAddressing/1(addr_r) -> Low_Gain_Table/4(rd_addr), Unit Delay3/1, Subtract/1  "addr_low"
  Abs/1 -> Unit Delay2/1, LogAddressing/1(x_in)  "|X_in|"
  Data_In/1 -> Abs/1
  Constant/1 -> Subtract/2
  Subtract/1 -> High_Gain_Table/4(rd_addr)  "addr_high"
  Low_Gain_Table/1(wr_dout) -> Terminator/1
  High_Gain_Table/1(wr_dout) -> Terminator1/1
  High_Gain_Table/2(rd_dout) -> Linear_Approximation/1(G_high)  "G_high"
  Low_Gain_Table/2(rd_dout) -> Linear_Approximation/2(G_low)  "G_low"
  Linear_Approximation/1(G_Desired) -> Gain_C_out/1
  Unit Delay2/1 -> Unit Delay1/1
  Unit Delay1/1 -> Linear_Approximation/4(|X_in|)
  Unit Delay3/1 -> Linear_Approximation/3(addr_low)

== system sm_DynamicCompressionOLD/SG_DataPlane/Avalon Data Processing/Left Channel Processing/recalculate/Nchan_FbankAGC_AID/Compression_5/Compression_Envelope ==
  note: Curr > Desired:
      | Attack
  note: Curr < Desired:
      | Release
  Desired_Gain : Inport
  Curr_Gain : Inport  Port=2
  Attack_Envelope : Subsystem  TreatAsAtomicUnit=on
  Compare To Zero : simulink/Logic and Bit Operations/Compare To Zero  relop=>=  OutDataTypeStr=boolean
  Logical Operator : Logic  Operator=NOT  AllPortsSameDT=off  OutDataTypeStr=boolean
  Release_Envelope : Subsystem  TreatAsAtomicUnit=on
  Subtract : Sum  Inputs=-+  AccumDataTypeStr=fixdt(1,W_bits,F_bits)  OutDataTypeStr=Inherit: Same as accumulator
  Switch : Switch
  Gain_Out : Outport
  wires:
  Desired_Gain/1 -> Attack_Envelope/2(Desired), Release_Envelope/2(Desired), Subtract/1
  Curr_Gain/1 -> Attack_Envelope/1(Curr), Subtract/2, Release_Envelope/1(Curr)
  Subtract/1 -> Switch/2, Compare To Zero/1
  Compare To Zero/1 -> Attack_Envelope/Enable, Logical Operator/1
  Logical Operator/1 -> Release_Envelope/Enable
  Switch/1 -> Gain_Out/1
  Attack_Envelope/1(Gain_out) -> Switch/1
  Release_Envelope/1(Gain_out) -> Switch/3
